simulink model "hw32f2"  (R2017a)
settings: Solver=VariableStepAuto  StartTime=0.0  StopTime=10.0  RelTol=1e-3
undefined symbols (not defined in the file): sigbuilder_block
settings Model: Creator=Soutrik  LastModifiedBy=Soutrik

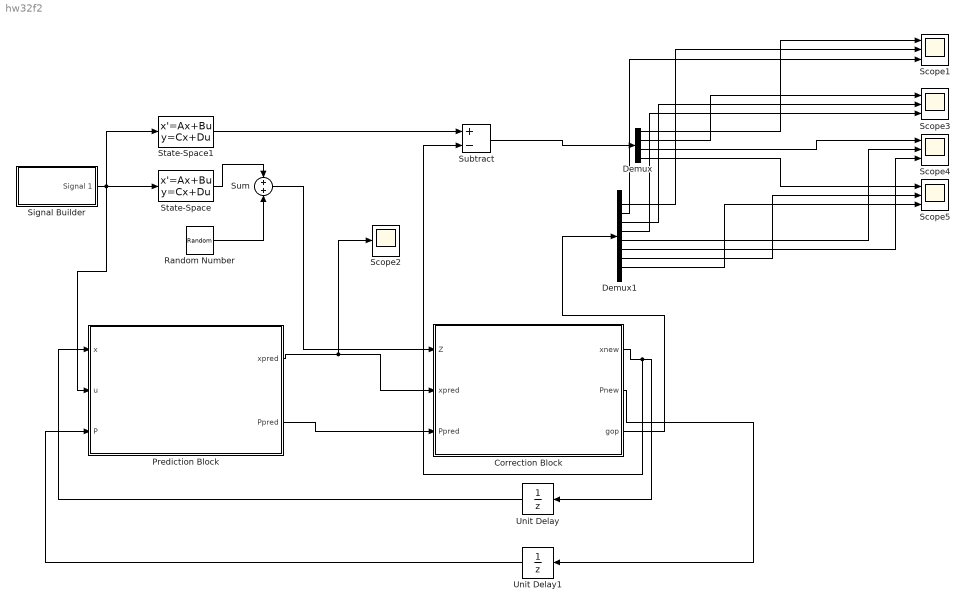
== system hw32f2 ==
  Correction Block : MATLAB Function  TreatAsAtomicUnit=on
  Demux : Demux
  Demux1 : Demux  Outputs=8
  Prediction Block : MATLAB Function  TreatAsAtomicUnit=on
  Random Number : RandomNumber  Variance=[0.0001, 0.0000001, 0.00002, 0.00002]  SampleTime=0.01
  Scope{1,3..5} (4 alike) : Scope  NumInputPorts=3
  Scope2 : Scope
  Signal Builder : Subsystem  Tag=STV Subsys  LoadFcn=sigbuilder_block('load');  StartFcn=sigbuilder_block('start');  StopFcn=sigbuilder_block('stop');  ClipboardFcn=sigbuilder_block('clipboard');  mask(Sigbuilder block){tuvar=[0:10]}
      mask help: Simulink:masks:SigbuilderBlock_MD
      mask init:
      | if ~strcmp(get_param(bdroot(gcbh),'SimulationStatus'),'stopped') tuvar = sigbuilder_block('maskInit'); end
      settings: CopyFcn=sigbuilder_block('copy');  DeleteFcn=sigbuilder_block('delete');  ModelCloseFcn=sigbuilder_block('modelClose');  PreSaveFcn=sigbuilder_block('preSave');  PauseFcn=sigbuilder_block('pause');  ContinueFcn=sigbuilder_block('continue');  NameChangeFcn=sigbuilder_block('namechange');  OpenFcn=sigbuilder_block('open',[300 184.875 550.5 400.125 ]);  CloseFcn=sigbuilder_block('close');
      mask Display: plot(0, 0, 100, 100,[2, 2, 32, 32, 2], [68, 8, 8, 68, 68],[32, 2], [38, 38], [32, 19, 2],[53, 60, 44], [32, 17, 17, 2],[16, 16, 31, 31]);txt = getActiveGroup(gcbh);text(2, 100, txt,'verticalAlignment', 'top');
  State-Space : StateSpace  A=|  B=|  C=|  D=[0;0;0;0];  X0=0
      A=|
      | [0 1.0000 0 0;
      | 0 -0.9965 0 -0.3000;
      | -0.3197 -0.5176 -0.0100 -0.7000;
      | 0 0 -0.0005 -0.9924];
      B=|
      | [ 0;
      | -0.0013;
      | 0.0001;
      | -0.0201];
      C=|
      | [0 0 0.9963 0.0862;
      | 0 0 -0.0001 0.0017;
      | 1.0000 0 0 0;
      | 0 1.0000 0 0];
  State-Space1 : StateSpace  A=|  B=|  C=[1 0 0 0;0 1 0 0;0 0 1 0;0 0 0 1]  D=[0;0;0;0];  X0=0
      A=|
      | [0 1.0000 0 0;
      | 0 -0.9965 0 -0.3000;
      | -0.3197 -0.5176 -0.0100 -0.7000;
      | 0 0 -0.0005 -0.9924];
      B=|
      | [ 0;
      | -0.0013;
      | 0.0001;
      | -0.0201];
  Subtract : Sum  Inputs=+-
  Sum : Sum  Inputs=2
  Unit Delay : UnitDelay  SampleTime=-1
  Unit Delay1 : UnitDelay  SampleTime=-1
  wires:
  Prediction Block/1(xpred) -> Scope2/1, Correction Block/2(xpred)
  State-Space/1 -> Sum/1
  Random Number/1 -> Sum/2
  Signal Builder/1(Signal 1) -> State-Space1/1, Prediction Block/2(u), State-Space/1
  Correction Block/1(xnew) -> Subtract/2, Unit Delay/1
  Correction Block/2(Pnew) -> Unit Delay1/1
  Prediction Block/2(Ppred) -> Correction Block/3(Ppred)
  Sum/1 -> Correction Block/1(Z)
  Unit Delay/1 -> Prediction Block/1(x)
  Unit Delay1/1 -> Prediction Block/3(P)
  State-Space1/1 -> Subtract/1
  Subtract/1 -> Demux/1
  Demux/1 -> Scope1/1
  Demux/2 -> Scope3/1
  Demux/3 -> Scope4/1
  Demux/4 -> Scope5/1
  Demux1/1 -> Scope1/2
  Demux1/2 -> Scope1/3
  Demux1/3 -> Scope3/2
  Demux1/4 -> Scope3/3
  Demux1/5 -> Scope4/2
  Demux1/6 -> Scope4/3
  Demux1/7 -> Scope5/2
  Demux1/8 -> Scope5/3
  Correction Block/3(gop) -> Demux1/1

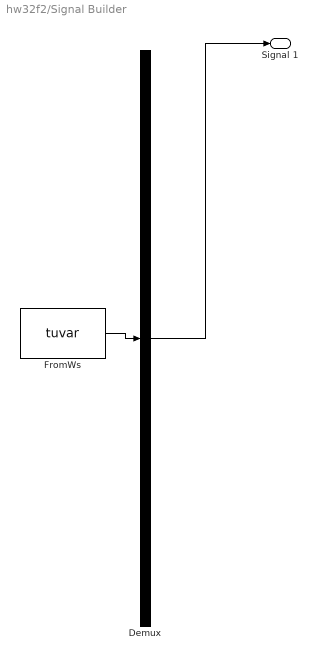
== system hw32f2/Signal Builder ==
  Demux : Demux  Tag=STV Demux  Outputs=1
  FromWs : FromWorkspace  Tag=STV FromWs  VariableName=tuvar  SampleTime=0
      SigBuilderData=|
      | common.afterFinalStr = 'Extrapolate'
      | common.sampleTime = 0
      | dataSet.timeRange = [0 10]
      | dataSet.name = 'Group 1'
      | sbobj.Groups.Name = 'Group 1'
      | sbobj.Groups.Signals.Name = 'Signal 1'
      | sbobj.Groups.Signals.XData = [0 1.02 1.02 2.04 2.04 3.04 3.04 10]
      | sbobj.Groups.Signals.YData = [0 -0.002 50 50 -50 -50 0 0]
  Signal 1 : Outport  Tag=STV Outport
  wires:
  Demux/1 -> Signal 1/1
  FromWs/1 -> Demux/1

== matlab function hw32f2/Correction Block ==
  data: Z input; xnew output; xpred input; Ppred input; Pnew output; gop output
function [xnew, Pnew,gop] = corrector(Z,xpred,Ppred)
%xpred= A*x+B*U;
%Ppred=A*P*A'+Q;
xnew=zeros(4,1);
Pnew=zeros(4);
gop=zeros(8,1);
R=diag([0.0001, 0.0000001, 0.00002, 0.00002]);
c = [0 0 0.9963 0.0862;
0 0 -0.0001 0.0017;
1.0000 0 0 0;
0 1.0000 0 0];
H=c;
K=Ppred*transpose(H)*inv(H*Ppred*(H)'+R);
Pnew=((eye(4)-K*H)*Ppred*transpose(eye(4)-K*H))+K*R*transpose(K);
xnew=xpred+K*(Z-H*xpred);

P44=Pnew(4,4)
gop(8,1)=sqrt(P44);
gop(7,1)=-sqrt(P44);
P33=Pnew(3,3)
gop(6,1)=sqrt(P33);
gop(5,1)=-sqrt(P33);
P22=Pnew(2,2)
gop(4,1)=sqrt(P22);
gop(3,1)=-sqrt(P22);
P11=Pnew(1,1)
gop(2,1)=sqrt(P11);
gop(1,1)=-sqrt(P11);

end

== matlab function hw32f2/Prediction Block ==
  data: x input; u input; xpred output; P input; Ppred output
function [xpred, Ppred] = predict(x, u, P)
%xpred= A*x+B*U;
%Ppred=A*P*A'+Q;
xpred=zeros(4,1);
Ppred=zeros(4);
b = [ 0;-0.0013;0.0001;-0.0201];
a =[0 1.0000 0 0;0 -0.9965 0 -0.3000;-0.3197 -0.5176 -0.0100 -0.7000;0 0 -0.0005 -0.9924];
Q =100*eye(4);
P=eye(4);
Ad=expm(a*0.01);
Bd=inv(a)*(Ad-eye(4))*b;
F=[-a Q;zeros(4,4) a'];
G=expm(F*0.01);
GLr=G(5:8,5:8);
Gur=G(1:4,5:8);
Qd=GLr'*Gur;
xpred=Ad*x+Bd*u;
Ppred=Ad*P*Ad'+Qd;

end
